simulink model "ClosedLoopControl"  (R2016b)
settings: Solver=FixedStepDiscrete  StartTime=0.0  StopTime=Inf  FixedStep=sCoreParams.core.stepPeriod  RelTol=1e-3  EnableMultiTasking=on
undefined symbols (not defined in the file): fdesignblkfcn, gcbh, High, sCoreParams, sCoreParams_decoders_chanceDetector_randStimEventsPerSec, sCoreParams_decoders_txDetector_channel1, sCoreParams_decoders_txDetector_channel2, sCoreParams_decoders_txDetector_detectChannelInds, sCoreParams_decoders_txDetector_nChannels, sCoreParams_Features_Baseline_initialThresholdValue, sCoreParams_Features_Baseline_weightPreviousThreshold, sCoreParams_Features_Data_SmoothWindowsDurationSamples, sCoreParams_stimulator_stimAfterDelaySteps
libraries: dsparch4 x20, dspstat3 x19, dspspect3 x6, dspfdesign x2, dspindex x2, dspswit3 x1
(part 2 of 6)

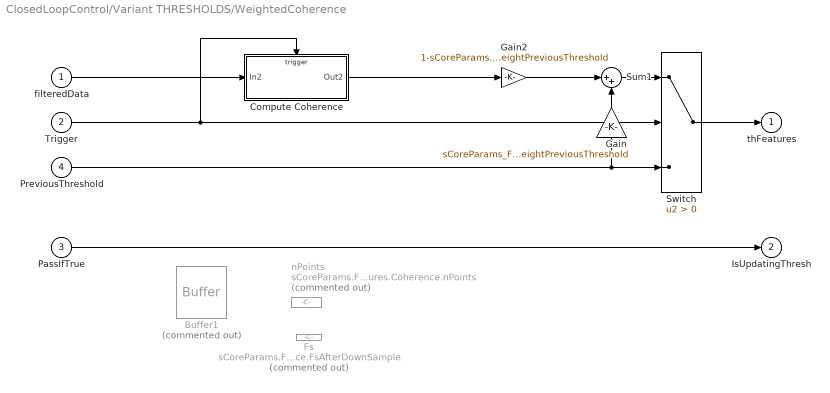
== system ClosedLoopControl/Variant THRESHOLDS/WeightedCoherence ==
  filteredData : Inport  SampleTime=sCoreParams.core.stepPeriod
  Trigger : Inport  Port=2  SampleTime=sCoreParams.core.stepPeriod
  PassIfTrue : Inport  Port=3  SampleTime=sCoreParams.core.stepPeriod
  PreviousThreshold : Inport  Port=4  SampleTime=sCoreParams.core.stepPeriod
  Buffer1 : Buffer  Commented=on  N=max(1, sCoreParams.Features.Coherence.WindowDurationSec - sCoreParams.Features.Baseline.durationSec)  V="max(0, sCoreParams.Features.Coherence.WindowDurationSec - sCoreParams.Features.Baseline.durationSec  -1)"  TreatMby1Signals=One channel
  Compute Coherence : Subsystem  TreatAsAtomicUnit=on
  Fs : Constant  Commented=on  Value=sCoreParams.Features.Coherence.FsAfterDownSample
  Gain : Gain  Gain=sCoreParams_Features_Baseline_weightPreviousThreshold  OutDataTypeStr=Inherit: Same as input
  Gain2 : Gain  Gain=1-sCoreParams.Features.Baseline.weightPreviousThreshold
  Sum1 : Sum  Inputs=|++
  Switch : Switch  Criteria=u2 > Threshold  InputSameDT=on
  nPoints : Constant  Commented=on  Value=sCoreParams.Features.Coherence.nPoints
  thFeatures : Outport  SampleTime=sCoreParams.core.stepPeriod
  IsUpdatingThresh : Outport  Port=2  SampleTime=sCoreParams.core.stepPeriod
  wires:
  PassIfTrue/1 -> IsUpdatingThresh/1
  Trigger/1 -> Compute Coherence/Trigger, Switch/2
  Gain/1 -> Sum1/2
  PreviousThreshold/1 -> Switch/3, Gain/1
  Sum1/1 -> Switch/1
  Switch/1 -> thFeatures/1
  filteredData/1 -> Compute Coherence/1(In2)
  Compute Coherence/1(Out2) -> Gain2/1
  Gain2/1 -> Sum1/1

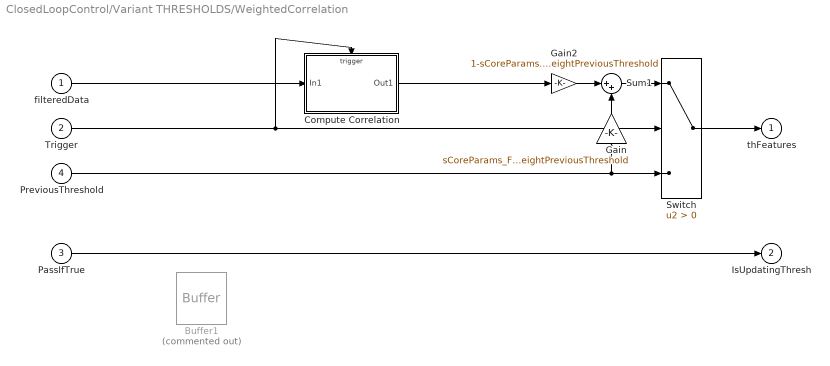
== system ClosedLoopControl/Variant THRESHOLDS/WeightedCorrelation ==
  filteredData : Inport  SampleTime=sCoreParams.core.stepPeriod
  Trigger : Inport  Port=2  SampleTime=sCoreParams.core.stepPeriod
  PassIfTrue : Inport  Port=3  SampleTime=sCoreParams.core.stepPeriod
  PreviousThreshold : Inport  Port=4  SampleTime=sCoreParams.core.stepPeriod
  Buffer1 : Buffer  Commented=on  N=max(1, sCoreParams.Features.Coherence.WindowDurationSec - sCoreParams.Features.Baseline.durationSec)  V="max(0, sCoreParams.Features.Coherence.WindowDurationSec - sCoreParams.Features.Baseline.durationSec  -1)"  TreatMby1Signals=One channel
  Compute Correlation : Subsystem
  Gain : Gain  Gain=sCoreParams_Features_Baseline_weightPreviousThreshold  OutDataTypeStr=Inherit: Same as input
  Gain2 : Gain  Gain=1-sCoreParams.Features.Baseline.weightPreviousThreshold
  Sum1 : Sum  Inputs=|++
  Switch : Switch  Criteria=u2 > Threshold  InputSameDT=on
  thFeatures : Outport  SampleTime=sCoreParams.core.stepPeriod
  IsUpdatingThresh : Outport  Port=2  SampleTime=sCoreParams.core.stepPeriod
  wires:
  PassIfTrue/1 -> IsUpdatingThresh/1
  Trigger/1 -> Compute Correlation/Trigger, Switch/2
  Gain/1 -> Sum1/2
  Gain2/1 -> Sum1/1
  PreviousThreshold/1 -> Switch/3, Gain/1
  Sum1/1 -> Switch/1
  Switch/1 -> thFeatures/1
  filteredData/1 -> Compute Correlation/1(In1)
  Compute Correlation/1(Out1) -> Gain2/1

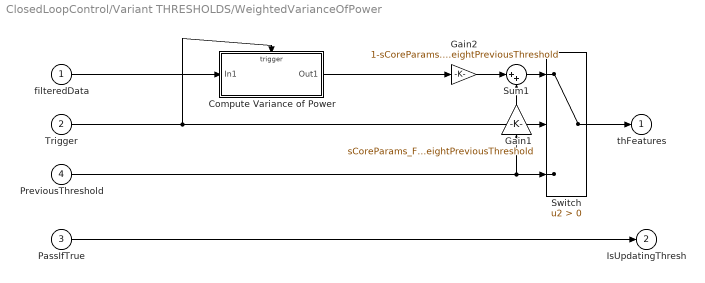
== system ClosedLoopControl/Variant THRESHOLDS/WeightedVarianceOfPower ==
  filteredData : Inport  SampleTime=sCoreParams.core.stepPeriod
  Trigger : Inport  Port=2  SampleTime=sCoreParams.core.stepPeriod
  PassIfTrue : Inport  Port=3  SampleTime=sCoreParams.core.stepPeriod
  PreviousThreshold : Inport  Port=4  SampleTime=sCoreParams.core.stepPeriod
  Compute Variance of Power : Subsystem  TreatAsAtomicUnit=on
  Gain1 : Gain  Gain=sCoreParams_Features_Baseline_weightPreviousThreshold
  Gain2 : Gain  Gain=1-sCoreParams.Features.Baseline.weightPreviousThreshold
  Sum1 : Sum  Inputs=|++
  Switch : Switch  Criteria=u2 > Threshold  InputSameDT=on
  thFeatures : Outport  SampleTime=sCoreParams.core.stepPeriod
  IsUpdatingThresh : Outport  Port=2  SampleTime=sCoreParams.core.stepPeriod
  wires:
  PassIfTrue/1 -> IsUpdatingThresh/1
  Trigger/1 -> Compute Variance of Power/Trigger, Switch/2
  Gain1/1 -> Sum1/2
  Sum1/1 -> Switch/1
  PreviousThreshold/1 -> Gain1/1, Switch/3
  Switch/1 -> thFeatures/1
  Gain2/1 -> Sum1/1
  filteredData/1 -> Compute Variance of Power/1(In1)
  Compute Variance of Power/1(Out1) -> Gain2/1

== system ClosedLoopControl/FilterBanks/Variant FILTER 1000/12-16HZ Spindles IIR ==
  EEGData : Inport
  Generated Filter Block : dsparch4/Biquad Filter  Tag=BlockMethodSubSystem  IIRFiltStruct=Direct form II  CoeffSource=Specify via dialog  BiQuadCoeffs=[0.01746549245317567 0 -0.01746549245317567 1 -1.9705415096766299 0.97705698823686593;0.0038937137359003394 0 -0.0038937137359003394 1 -1.9650909272804944 0.97368290679133707;0.031007791735965635 0 -0.031007791735965635 1 -1.9892481031485743 0.99479646997826532;0.018203868513229925 0 -0.018203868513229925 1 -1.9826474461497503 0.99292534324006443;0.0075528901021054973 0 -0.0075528901021054973 1 -1.9652250202332286 0.97269707225051594;0.026672977850967713 0 -0.026672977850967713 1 -1.9791288468533708 0.984990002041639;2 0 -2 1 -1.971173083664119 0.98079635113195673]  a0Flag=Warning  IC=0  ICnum=0  ICden=0  InputProcessing=Columns as channels (frame based)  denAccumFracLength=30  denProdOutputFracLength=30  secondMemoryFracLength=15  roundingMode=Floor  overflowMode=off  ScaleValues=[0.0018422414087593609;1;1;1;1;1;1;3.2084067595505501]  optimizeScaleValues=off  ScaleValueMode=Specify via input port (g)  scaleValueFracLength=14  FilterSource=Specify via dialog  FilterObject=BQF
  filteredData : Outport
  wires:
  EEGData/1 -> Generated Filter Block/1
  Generated Filter Block/1 -> filteredData/1

== system ClosedLoopControl/FilterBanks/Variant FILTER 1000/140-200Hz Ripple IIR ==
  EEGData : Inport
  Generated Filter Block : dsparch4/Biquad Filter  Tag=BlockMethodSubSystem  IIRFiltStruct=Direct form II  CoeffSource=Specify via dialog  BiQuadCoeffs=[0.21787375026202307 0 -0.21787375026202307 1 -0.96331857763445794 0.69801532319874404;0.058284123788188938 0 -0.058284123788188938 1 -0.67658046347367318 0.67021424663244811;0.42901503492070636 0 -0.42901503492070636 1 -1.2441636826365454 0.92340693897894432;0.23149664116898019 0 -0.23149664116898019 1 -0.56087223186376556 0.90493867584787147;0.10425613493575765 0 -0.10425613493575765 1 -0.81058602955415293 0.6527706279240969;0.34638405047355492 0 -0.34638405047355492 1 -1.1125181562081008 0.79248495781259809;0.62838189778108478 0 -0.62838189778108478 1 -0.58620830873583829 0.75565502116544325]  a0Flag=Warning  IC=0  ICnum=0  ICden=0  InputProcessing=Columns as channels (frame based)  denAccumFracLength=30  denProdOutputFracLength=30  secondMemoryFracLength=15  roundingMode=Floor  overflowMode=off  ScaleValues=[0.24674852863293925;1;1;1;1;1;1;1]  optimizeScaleValues=off  ScaleValueMode=Specify via input port (g)  scaleValueFracLength=14  FilterSource=Specify via dialog  FilterObject=BQF
  filteredData : Outport
  wires:
  EEGData/1 -> Generated Filter Block/1
  Generated Filter Block/1 -> filteredData/1

== system ClosedLoopControl/FilterBanks/Variant FILTER 1000/145-200Hz Ripple FIR ==
  EEGData : Inport
  Generated Filter Block : DiscreteFir  Tag=BlockMethodSubSystem  Coefficients=[-0.030781520603345755 0.029736587613204871 0.016279349881715796 0.0078304734697767775 0.0034101124575861563 0.0021109050937578866 0.0029359501791036482 0.0048221357516104943 0.0066675765400677559 0.0075439573200530088 0.0068299029664432159 0.0044170245691875151 0.0007305503624317547 -0.0033144418142821638 -0.0066073626352400397 -0.008115382277290431 -0.007299157247865555 -0.0042500768030829042 0.0001902291282893237 0.0047615272618279983 0.0080537753119725719 0.0090888577269477855 0.007501544338330314 0.0038465594631155176 -0.00074048500280713553 -0.0048863103096512331 -0.0072169181698771429 -0.0073994531081829351 -0.0054270557962657132 -0.002254737434171504 0.00086546613635283404 0.0029149802832981117 0.0034583853146492802 0.0026234557641752754 0.001164732411809373 5.1783863659192464e-05 2.3369551283396184e-05 0.0011599107816354856 0.0028744791094547709 0.004135969419948364 0.0039639887525646025 0.0018331530274210903 -0.0019498921461991101 -0.0062991090714655182 -0.0096028435909793972 -0.010407292076703323 -0.0079421078421768043 -0.0026102640831030394 0.0041590394472750397 0.010237281364097572 0.013611983265214941 0.013116126210911384 0.0087781592628307439 0.0020124063186148997 -0.005021276797438759 -0.010123284187206115 -0.011821380571436675 -0.0099304545038921554 -0.0055932597013606603 -0.00071349819259146352 0.0028002388976299947 0.0038275185978517978 0.0025285946144394666 0.00024688745347431484 -0.0011164507549987698 -3.8298925510396598e-05 0.0038051022729689021 0.00918952477604211 0.013626718379269272 0.014320948674260946 0.009371767654852238 -0.0011215127004242931 -0.014722781888086886 -0.02711168652799726 -0.033490181243977103 -0.030255934127276694 -0.016584097409115692 0.0047929614203095217 0.02810395806549059 0.046075325861400326 0.052266726383597022 0.04336162944653018 0.020556639691233745 -0.010420977616046684 -0.040753154116921785 -0.06119608459496325 -0.065000080365273327 -0.050152269558981596 -0.020277362294476072 0.016311587571896234 0.049020798279318864 0.068226011237433576 0.068226011237433576 0.049020798279318864 0.016311587571896234 -0.020277362294476072 -0.050152269558981596 -0.065000080365273327 -0.06119608459496325 -0.040753154116921785 -0.010420977616046684 0.020556639691233745 0.04336162944653018 0.052266726383597022 0.046075325861400326 0.02810395806549059 0.0047929614203095217 -0.016584097409115692 -0.030255934127276694 -0.033490181243977103 -0.02711168652799726 -0.014722781888086886 -0.0011215127004242931 0.009371767654852238 0.014320948674260946 0.013626718379269272 0.00918952477604211 0.0038051022729689021 -3.8298925510396598e-05 -0.0011164507549987698 0.00024688745347431484 0.0025285946144394666 0.0038275185978517978 0.0028002388976299947 -0.00071349819259146352 -0.0055932597013606603 -0.0099304545038921554 -0.011821380571436675 -0.010123284187206115 -0.005021276797438759 0.0020124063186148997 0.0087781592628307439 0.013116126210911384 0.013611983265214941 0.010237281364097572 0.0041590394472750397 -0.0026102640831030394 -0.0079421078421768043 -0.010407292076703323 -0.0096028435909793972 -0.0062991090714655182 -0.0019498921461991101 0.0018331530274210903 0.0039639887525646025 0.004135969419948364 0.0028744791094547709 0.0011599107816354856 2.3369551283396184e-05 5.1783863659192464e-05 0.001164732411809373 0.0026234557641752754 0.0034583853146492802 0.0029149802832981117 0.00086546613635283404 -0.002254737434171504 -0.0054270557962657132 -0.0073994531081829351 -0.0072169181698771429 -0.0048863103096512331 -0.00074048500280713553 0.0038465594631155176 0.007501544338330314 0.0090888577269477855 0.0080537753119725719 0.0047615272618279983 0.0001902291282893237 -0.0042500768030829042 -0.007299157247865555 -0.008115382277290431 -0.0066073626352400397 -0.0033144418142821638 0.0007305503624317547 0.0044170245691875151 0.0068299029664432159 0.0075439573200530088 0.0066675765400677559 0.0048221357516104943 0.0029359501791036482 0.0021109050937578866 0.0034101124575861563 0.0078304734697767775 0.016279349881715796 0.029736587613204871 -0.030781520603345755]  InputProcessing=Columns as channels (frame based)
  filteredData : Outport
  wires:
  EEGData/1 -> Generated Filter Block/1
  Generated Filter Block/1 -> filteredData/1

== system ClosedLoopControl/FilterBanks/Variant FILTER 1000/15-30Hz Beta FIR ==
  EEGData : Inport
  Generated Filter Block : DiscreteFir  Tag=BlockMethodSubSystem  Coefficients=[0.00024932604967076838 0.00022562835097991477 0.00020055883023604209 0.00017450536010432124 0.00014787470676203059 0.00012108823390752595 9.4577357124501601e-05 6.8778794034300684e-05 4.4129658786645323e-05 2.1062452077078791e-05 -2.7492423039110665e-19 -1.8649603383242571e-05 -3.4497993888248867e-05 -4.7181419195105332e-05 -5.6365448928950234e-05 -6.1749457622014875e-05 -6.3070826807644178e-05 -6.0108814576680591e-05 -5.2688043611973456e-05 -4.0681561988766557e-05 -2.401343486143125e-05 -2.6608295179705497e-06 2.3344438865809144e-05 5.3914928145513692e-05 8.8907178484600832e-05 0.00012812192564416256 0.00017130492763639147 0.00021814840757232323 0.00026829310886882917 0.00032133095223859563 0.0003768082771425536 0.00043422964371071202 0.00049306216460859417 0.00055274033001634403 0.00061267128286881189 0.00067224049584787074 0.00073081779639075947 0.00078776368124497246 0.00084243585792020525 0.00089419594681682153 0.00094241627489654754 0.00098648668954764637 0.0010258213198195128 0.0010598652114882623 0.0010881007624864356 0.0011100538860983283 0.0011252998309913629 0.0011334685896186197 0.0011342498297744687 0.0011273972880916526 0.0011127325690035576 0.0010901482981200605 0.0010596105850321073 0.0010211607572136851 0.0009749163338677976 0.00092107121619643812 0.00085989507858800552 0.0007917319535292195 0.00071699801157699126 0.000636178546380586 0.00054982418343449066 0.00045854633987444526 0.00036301197110909526 0.00026393764831425211 0.00016208301871255902 5.8243708028869324e-05 -4.6756268537101536e-05 -0.00015207251412670736 -0.00025684859845693733 -0.00036022466317640564 -0.00046134619693138701 -0.00055937288948681779 -0.00065348747192239289 -0.00074290444855744885 -0.00082687862588018109 -0.00090471334438626367 -0.00097576832087874178 -0.0010394670114429023 -0.0010953034089747223 -0.0011428481937856628 -0.0011817541613957556 -0.0012117608581163283 -0.0012326983623577709 -0.001244490157711635 -0.0012471550526754304 -0.0012408081113295473 -0.0012256605692480087 -0.0012020187193297893 -0.0011702817629714256 -0.0011309386329549156 -0.0010845638054844833 -0.001031812129855466 -0.0009734127151604698 -0.00091016192411399002 -0.00084291553438961802 -0.00077258013769825561 -0.00070010385607981835 -0.00062646646342703839 -0.0005526690080073168 -0.0004797230386016781 -0.00040863954275302474 -0.00034041771043132122 -0.00027603364011376626 -0.00021642910678700521 -0.00016250051266128044 -0.00011508814141064184 -7.4965835499315943e-05 -4.2831213615604891e-05 -1.9296541418413303e-05 -4.8803637284107098e-06 -1.5115631016753627e-19 -4.9649974395269964e-06 -1.9971627550228426e-05 -4.5098502258702979e-05 -8.0303375196634768e-05 -0.00012542118227197094 -0.0001801633634729392 -0.00024411849502299244 -0.00031675424767009996 -0.00039742067318219532 -0.00048535480717015462 -0.00057968656231336378 -0.00067944587206669998 -0.00078357103112883036 -0.00089091816549832607 -0.0010002717519816938 -0.0011103560946900746 -0.0012198476545067958 -0.0013273881168597975 -0.0014315980735153974 -0.0015310911856396493 -0.0016244886881564714 -0.00171043408956193 -0.0017876079169135538 -0.0018547423527700514 -0.0019106356094641382 -0.0019541658862868043 -0.0019843047569679832 -0.0020001298382613876 -0.0020008365954695844 -0.0019857491473510187 -0.0019543299409892647 -0.0019061881768149373 -0.0018410868749752605 -0.001758948486552175 -0.0016598589666296502 -0.0015440702407827466 -0.0014120010120704913 -0.0012642358719159457 -0.0011015226951933369 -0.00092476831724877333 -0.00073503250828539982 -0.00053352027836815253 -0.0003215725640653392 -0.00010065536526088647 0.00012765258224192586 0.00036167349622888341 0.00059964548191373797 0.00083973857760329443 0.0010800717660899655 0.0013187307933636354 0.0015537866253548353 0.0017833143641044383 0.0020054124371196732 0.0022182218678259581 0.0024199454310448224 0.0026088664953892731 0.0027833673544188494 0.002941946850368166 0.0030832370982642947 0.0032060191242710254 0.0033092372401093842 0.00339201198535369 ...(+10128 chars)]  InputProcessing=Columns as channels (frame based)
  filteredData : Outport
  wires:
  EEGData/1 -> Generated Filter Block/1
  Generated Filter Block/1 -> filteredData/1

== system ClosedLoopControl/FilterBanks/Variant FILTER 1000/15-30Hz Beta IIR ==
  EEGData : Inport
  Generated Filter Block : dsparch4/Biquad Filter  Tag=BlockMethodSubSystem  IIRFiltStruct=Direct form II  CoeffSource=Specify via dialog  BiQuadCoeffs=[0.066223099366740951 0 -0.066223099366740951 1 -1.9198928964135957 0.95434199780108331;0.056467648873273713 0 -0.056467648873273713 1 -1.9351997380399308 0.94559569189292736;0.048139705930922046 0 -0.048139705930922046 1 -1.8793203951971771 0.89972224210887464;0.052012688134885021 0 -0.052012688134885021 1 -1.9022753798144565 0.91633139369780681;0.018466663590485453 0 -0.018466663590485453 1 -1.8833214970678875 0.91147221732826511;0.047917488571810593 0 -0.047917488571810593 1 -1.9836338187702465 0.99220535429046763;0.068553596218735871 0 -0.068553596218735871 1 -1.9478187570894017 0.98406102288814179;0.035684596971190814 0 -0.035684596971190814 1 -1.9184287784120526 0.93033618287560638;0.064326690729456126 0 -0.064326690729456126 1 -1.8978501006004 0.92950796112203882;0.05426936542901882 0 -0.05426936542901882 1 -1.888440628376189 0.90535267359424354;0.068030209651796847 0 -0.068030209651796847 1 -1.8771813037252187 0.9014520972123361;0.035722451327353327 0 -0.035722451327353327 1 -1.9678787137562923 0.97669433626883684;2 0 -2 1 -1.9517590014341009 0.96115976859420349]  a0Flag=Warning  IC=0  ICnum=0  ICden=0  InputProcessing=Columns as channels (frame based)  denAccumFracLength=30  denProdOutputFracLength=30  secondMemoryFracLength=15  roundingMode=Floor  overflowMode=off  ScaleValues=[0.0084703427391639319;1;1;1;1;1;1;1;1;1;1;1;1;2.5495638182419023]  optimizeScaleValues=off  ScaleValueMode=Specify via input port (g)  scaleValueFracLength=14  FilterSource=Specify via dialog  FilterObject=BQF
  filteredData : Outport
  wires:
  EEGData/1 -> Generated Filter Block/1
  Generated Filter Block/1 -> filteredData/1

== system ClosedLoopControl/FilterBanks/Variant FILTER 1000/30-110Hz Gamma ==
  EEGData : Inport
  Generated Filter Block : dsparch4/Biquad Filter  Tag=BlockMethodSubSystem  IIRFiltStruct=Direct form II  CoeffSource=Specify via dialog  BiQuadCoeffs=[0.82943104360127162 0 -0.82943104360127162 1 -1.8183457880456473 0.86555013309266671;0.21351483903370441 0 -0.21351483903370441 1 -1.4410847446229762 0.83890122765295905;0.27245359693270271 0 -0.27245359693270271 1 -1.5352437473443921 0.63694019484137088;0.23741463270400096 0 -0.23741463270400096 1 -1.3380256330801488 0.62471192945933707;0.22171682131997325 0 -0.22171682131997325 1 -1.4036156937267288 0.57093225988445084;0.13338118805603641 0 -0.13338118805603641 1 -1.3621091572121378 0.56870830801771233;0.25173513791228957 0 -0.25173513791228957 1 -1.388153965891608 0.75109342907909371;0.25616838332127972 0 -0.25616838332127972 1 -1.6698296683378542 0.73629059356094473;0.049485114028227535 0 -0.049485114028227535 1 -1.9371437156763709 0.98054077689581631;0.28721409920587238 0 -0.28721409920587238 1 -1.51340629382632 0.94252833506192135;0.28185389458665555 0 -0.28185389458665555 1 -1.7740920325548135 0.82525504919152526;0.26200161383963994 0 -0.26200161383963994 1 -1.7252044629652221 0.78244434772121285;0.21765188776315755 0 -0.21765188776315755 1 -1.4637754333312696 0.59500984788338196;0.27041904886657164 0 -0.27041904886657164 1 -1.3405180456517258 0.5872964036840892;0.16097151831745662 0 -0.16097151831745662 1 -1.60628101900206 0.68680614711867571;0.29053184765179513 0 -0.29053184765179513 1 -1.3539378097971999 0.67956103690721736;0.10410147815491434 0 -0.10410147815491434 1 -1.8987522691133922 0.94231217905370779;2 0 -2 1 -1.8594926335496971 0.90427012472796742]  a0Flag=Warning  IC=0  ICnum=0  ICden=0  InputProcessing=Columns as channels (frame based)  denAccumFracLength=30  denProdOutputFracLength=30  secondMemoryFracLength=15  roundingMode=Floor  overflowMode=off  ScaleValues=[0.028522976766974045;1;1;1;1;1;1;1;1;1;1;1;1;1;1;1;1;1;1.1274493619551109]  optimizeScaleValues=off  ScaleValueMode=Specify via input port (g)  scaleValueFracLength=14  FilterSource=Specify via dialog  FilterObject=BQF
  filteredData : Outport
  wires:
  EEGData/1 -> Generated Filter Block/1
  Generated Filter Block/1 -> filteredData/1

== system ClosedLoopControl/FilterBanks/Variant FILTER 1000/30-55Hz LowGamma FIR ==
  EEGData : Inport
  Generated Filter Block : DiscreteFir  Tag=BlockMethodSubSystem  Coefficients=[0.012220426722110508 -0.012179228647942394 -0.0054004824998452744 -0.00086107993631961153 0.0018357528942907909 0.0031129006980230925 0.0033526002586839569 0.0029004097183938193 0.002025756039159722 0.00094619130244101926 -0.00019186502278131733 -0.0012796989292308341 -0.0022643735403191324 -0.0031100749332247601 -0.0038138220234182119 -0.0043728519036089321 -0.0048073661756172087 -0.0051211291794167951 -0.0053355515893745153 -0.0054503938965098165 -0.0054804722865874379 -0.0054225157087565935 -0.0052837766862496747 -0.0050558969555260557 -0.0047473427181577406 -0.0043490854638637624 -0.0038740240389517158 -0.0033141899320159045 -0.0026891371712456872 -0.0019988658326665788 -0.0012668077012148425 -0.00049777159136449409 0.00027980011654713644 0.0010569221711767803 0.0018012584862141282 0.0025073080725695955 0.0031419799261284092 0.0037039342557620781 0.0041592221536759701 0.00451661684396605 0.004753834670207643 0.004858091055885313 0.0048732693610234797 0.004719918151711854 0.004501106268126308 0.0041695525933403083 0.0037390943415244577 0.0032614183648101208 0.0027532787181978611 0.0022113037703167591 0.0016750315037899622 0.001183752691769548 0.00075535761814340149 0.00039953150366791961 0.00014046384937540252 6.1491868128734175e-06 1.1186901667634026e-05 0.00015526412697483837 0.0004330345318633678 0.00085176463289905009 0.0014052355878874233 0.0020800590767608707 0.002849623480313646 0.0036845580548849717 0.0045549014833176776 0.0054328429633881004 0.0062766851830694257 0.0070524883129054004 0.0077090516676290282 0.0082134484811023818 0.0085227769306376287 0.0086142017649426875 0.0084547786472301146 0.0080253554621038687 0.0073005963266854152 0.0062785521595116736 0.004954769987550566 0.0033487584764538918 0.0014699436712954949 -0.00064363377180517154 -0.0029663837162192072 -0.0054436946157823849 -0.0080298692849513926 -0.010667639233237229 -0.013277806853810465 -0.015812438746192266 -0.018188194707908951 -0.020345799993991307 -0.022224250296602483 -0.023753925738189897 -0.02488365206526176 -0.025570322564561061 -0.025766825493726914 -0.025444977817514449 -0.024595476521060467 -0.023213441870529743 -0.021305593868567389 -0.018898508751834929 -0.016029060137637101 -0.012740944050543842 -0.0090932386572889021 -0.0051505995714406739 -0.0009962643893293105 0.0032817393593285271 0.0076023297562782021 0.01187015497436876 0.01599167911755478 0.01987965668781326 0.023442825796413751 0.026611571958282988 0.029305287988366832 0.031470080206127349 0.033049785633532322 0.034015176943345569 0.034337823655261598 0.034015176943345569 0.033049785633532322 0.031470080206127349 0.029305287988366832 0.026611571958282988 0.023442825796413751 0.01987965668781326 0.01599167911755478 0.01187015497436876 0.0076023297562782021 0.0032817393593285271 -0.0009962643893293105 -0.0051505995714406739 -0.0090932386572889021 -0.012740944050543842 -0.016029060137637101 -0.018898508751834929 -0.021305593868567389 -0.023213441870529743 -0.024595476521060467 -0.025444977817514449 -0.025766825493726914 -0.025570322564561061 -0.02488365206526176 -0.023753925738189897 -0.022224250296602483 -0.020345799993991307 -0.018188194707908951 -0.015812438746192266 -0.013277806853810465 -0.010667639233237229 -0.0080298692849513926 -0.0054436946157823849 -0.0029663837162192072 -0.00064363377180517154 0.0014699436712954949 0.0033487584764538918 0.004954769987550566 0.0062785521595116736 0.0073005963266854152 0.0080253554621038687 0.0084547786472301146 0.0086142017649426875 0.0085227769306376287 0.0082134484811023818 0.0077090516676290282 0.0070524883129054004 0.0062766851830694257 0.0054328429633881004 0.0045549014833176776 0.0036845580548849717 0.002849623480313646 0.0020800590767608707 0.0014052355878874233 0.00085176463289905009 0.0004330345318633678 0.00015526412697483837 1.1186901667634026e-05 6.1491868128734175e-06 0.00014046384937540252 0.00039953150366791961 0.00075535761814340149 0.001183752691769548 0.0016750315037899622 0.0022113037703167591 ...(+1099 chars)]  InputProcessing=Columns as channels (frame based)
  filteredData : Outport
  wires:
  EEGData/1 -> Generated Filter Block/1
  Generated Filter Block/1 -> filteredData/1

== system ClosedLoopControl/FilterBanks/Variant FILTER 1000/30-55Hz LowGamma IIR ==
  EEGData : Inport
  Generated Filter Block : dsparch4/Biquad Filter  Tag=BlockMethodSubSystem  IIRFiltStruct=Direct form II  CoeffSource=Specify via dialog  BiQuadCoeffs=[0.10799779966567541 0 -0.10799779966567541 1 -1.8213059351723211 0.93080593354591523;0.087206628396552785 0 -0.087206628396552785 1 -1.8700150667203665 0.90983094754577998;0.079642318754869171 0 -0.079642318754869171 1 -1.7775727772918692 0.84640916667866339;0.075762671941351833 0 -0.075762671941351833 1 -1.8161028628727054 0.86693872891834445;0.033846832608554409 0 -0.033846832608554409 1 -1.7757901787287247 0.86644297049777186;0.065072203007372986 0 -0.065072203007372986 1 -1.9523142768092243 0.98658217881363142;0.054128178132898434 0 -0.054128178132898434 1 -1.8600871202136466 0.9756810586138418;0.10954509830118907 0 -0.10954509830118907 1 -1.7927016638303193 0.89360816778647045;0.10024430805902325 0 -0.10024430805902325 1 -1.8423311985853308 0.88678484220470721;0.082611886277899754 0 -0.082611886277899754 1 -1.7935496701663221 0.85258756197942498;0.11276238344522446 0 -0.11276238344522446 1 -1.7709985537539841 0.85065128142306534;0.065059502360374638 0 -0.065059502360374638 1 -1.9253364233492101 0.96024347511843622;2 0 -2 1 -1.8978656931910507 0.93457223452457516]  a0Flag=Warning  IC=0  ICnum=0  ICden=0  InputProcessing=Columns as channels (frame based)  denAccumFracLength=30  denProdOutputFracLength=30  secondMemoryFracLength=15  roundingMode=Floor  overflowMode=off  ScaleValues=[0.02285123356516695;1;1;1;1;1;1;1;1;1;1;1;1;1.286232826902199]  optimizeScaleValues=off  ScaleValueMode=Specify via input port (g)  scaleValueFracLength=14  FilterSource=Specify via dialog  FilterObject=BQF
  filteredData : Outport
  wires:
  EEGData/1 -> Generated Filter Block/1
  Generated Filter Block/1 -> filteredData/1
